simulink model "V0.2.4 - 2025-11-12 - FullFMS"  (R2025b)
settings: Solver=VariableStepAuto  StartTime=0.0  StopTime=inf  RelTol=1e-3
libraries: opcualib x2
(part 2 of 2)

== stateflow chart V0.2.4 - 2025-11-12 - FullFMS/Chart ==
  state VarDeclaration_20
    entry:
    %Control_20
    C_24_CRoute_In  = Control_20(1);
    C_25_CRoute_In  = Control_20(2);
    C_26_CRoute_In  = Control_20(3);
    C_27_CRoute_In  = Control_20(4);
    C_28_CRoute_In  = Control_20(5);
    C_29_CRoute_In  = Control_20(6);
    C_24_Request    = Control_20(7);
    C_24_CartDel    = Control_20(8);
    C_24_CRoute_Out = Control_20(9);
    C_25_Request    = Control_20(10);
    C_25_CartDel    = Control_20(11);
    C_25_CRoute_Out = Control_20(12);
    C_26_Request    = Control_20(13);
    C_26_CartDel    = Control_20(14);
    C_26_CRoute_Out = Control_20(15);
    C_27_Request    = Control_20(16);
    C_27_CartDel    = Control_20(17);
    C_27_CRoute_Out = Control_20(18);
    C_28_Request    = Control_20(19);
    C_28_CartDel    = Control_20(20);
    C_28_CRoute_Out = Control_20(21);
    C_29_Request    = Control_20(22);
    C_29_CartDel    = Control_20(23);
    C_29_CRoute_Out = Control_20(24);
    %Actuators_20
    F_22_Led_On       = Actuators_20(1);
    F_22_Led_Off      = Actuators_20(2);
    F_22_Conveyor   = Actuators_20(3);
    F_24_Release_FB   = Actuators_20(4);
    F_25_Release_FB   = Actuators_20(5);
    F_26_Release_FB   = Actuators_20(6);
    F_27_Release_FB   = Actuators_20(7);
    F_28_Release_FB   = Actuators_20(8);
    F_29_Release_FB   = Actuators_20(9);
    %Sensors_20
    O_20_On            = Sensors_20(1);
    O_20_Off           = Sensors_20(2);
    O_20_Controler_On  = Sensors_20(3);
    O_24_Cart_Stat     = Sensors_20(4);
    O_24_Cart_Next     = Sensors_20(5);
    O_24_Optic         = Sensors_20(6);
    O_24_Count         = Sensors_20(7);
    O_24_Pist_Bck      = Sensors_20(8);
    O_25_Cart_Stat     = Sensors_20(9);
    O_25_Cart_Next     = Sensors_20(10);
    O_25_Optic         = Sensors_20(11);
    O_25_Count         = Sensors_20(12);
    O_25_Pist_Back     = Sensors_20(13);
    O_26_Cart_Stat     = Sensors_20(14);
    O_26_Cart_Next     = Sensors_20(15);
    O_26_Optic         = Sensors_20(16);
    O_26_Count         = Sensors_20(17);
    O_26_Pist_Back     = Sensors_20(18);
    O_27_Cart_Stat     = Sensors_20(19);
    O_27_Cart_Next     = Sensors_20(20);
    O_27_Optic         = Sensors_20(21);
    O_27_Count         = Sensors_20(22);
    O_27_Pist_Back     = Sensors_20(23);
    O_28_Cart_Stat     = Sensors_20(24);
    O_28_Cart_Next     = Sensors_20(25);
    O_28_Optic         = Sensors_20(26);
    O_28_Count         = Sensors_20(27);
    O_28_Pist_Back     = Sensors_20(28);
    O_29_Cart_Stat     = Sensors_20(29);
    O_29_Cart_Next     = Sensors_20(30);
    O_29_Optic         = Sensors_20(31);
    O_29_Count         = Sensors_20(32);
    O_29_Pist_Back     = Sensors_20(33);
  state VarDeclaration_30
    entry:
    %AS_i_30
    A_34_Request    = AS_i_30(1);
    A_34_No_Cart    = AS_i_30(2);
    A_34_Cart_Full  = AS_i_30(3);
    A_34_CRoute_Out = AS_i_30(4);
    A_32_RoboCartID = AS_i_30(5);
    A_34_Cart_Stat  = AS_i_30(6);
    A_34_Cart_Next  = AS_i_30(7);
    A_34_Optic      = AS_i_30(8);
    A_34_Count      = AS_i_30(9);
    A_34_Pist_Bck   = AS_i_30(10);
    A_34_Release_FB = AS_i_30(11);
    A_34_CRoute_In  = AS_i_30(12);
    %Control_30
    C_30_Robot1   = Control_30(1);
    C_30_Robot2   = Control_30(2);
    C_35_Part_Del = Control_30(3);
    %Actuators_30
    F_33_Led_Start  = Actuators_30(1);
    F_33_Led_Reset  = Actuators_30(2);
    F_33_Led_Extra1 = Actuators_30(3);
    F_33_Led_Extra2 = Actuators_30(4);
    F_33_Spring_Cyl = Actuators_30(5);
    F_33_Cover_Cyl  = Actuators_30(6);
    %Sensors_30
    O_31_Start        = Sensors_30(1);
    O_31_Stop         = Sensors_30(2);
    O_31_Reset        = Sensors_30(3);
    O_31_Part_in_Claw = Sensors_30(4);
    O_31_Orientation  = Sensors_30(5);
    O_32_Sp_Cyl_Bck   = Sensors_30(6);
    O_32_Sp_Cyl_Fwd   = Sensors_30(7);
    O_32_Co_Cyl_Bck   = Sensors_30(8);
    O_32_Co_Cyl_Fwd   = Sensors_30(9);
    O_32_Sp_PickUp    = Sensors_30(10);
    O_32_Co_PickUp    = Sensors_30(11);
    O_32_CoMag_Empty  = Sensors_30(12);
  state VarDeclaration_40
    entry:
    %AS_i_40
    %Control_40
    %Actuators_40
    %Sensors_40
  state VarDeclaration_50
    entry:
    %AS_i_50
    A_54_Request    = AS_i_50(1);
    A_54_No_Cart    = AS_i_50(2);
    A_54_Cart_Full  = AS_i_50(3);
    A_54_CRoute_Out = AS_i_50(4);
    A_53_SortCartID = AS_i_50(5);
    A_54_Cart_Stat  = AS_i_50(6);
    A_54_Cart_Next  = AS_i_50(7);
    A_54_Optic      = AS_i_50(8);
    A_54_Count      = AS_i_50(9);
    A_54_Pist_Bck   = AS_i_50(10);
    A_54_Release_FB = AS_i_50(11);
    A_54_CRoute_In  = AS_i_50(12);
    C_55_Start      = AS_i_50(13);
    C_55_Cart2Del   = AS_i_50(14);
    %Control_50
    C_55_Initialization = Control_50(1);
    C_55_PD_Sort        = Control_50(2);
    C_52_Profibus       = Control_50(3);
    C_55_Start          = Control_50(4);
    C_55_Cart2Del       = Control_50(5);
    %Actuators_50
    F_52_Claw_2_Del  = Actuators_50(1);
    F_52_Claw_2_Cart = Actuators_50(2);
    F_52_Claw_Down   = Actuators_50(3);
    F_52_Close_Claw  = Actuators_50(4);
    F_53_Led_Start   = Actuators_50(5);
    F_53_Led_Reset   = Actuators_50(6);
    F_53_Led_Extra1  = Actuators_50(7);
    F_53_Led_Extra2  = Actuators_50(8);
    F_53_Panel_O4    = Actuators_50(9);
    F_53_Panel_O5    = Actuators_50(10);
    F_53_Panel_O6    = Actuators_50(11);
    F_53_Panel_O7    = Actuators_50(12);
    %Sensors_50
    O_50_Part_Reserve = Sensors_50(1);
    O_50_Claw_Cart    = Sensors_50(2);
    O_50_Claw_Del     = Sensors_50(3);
    O_50_Claw_Reserve = Sensors_50(4);
    O_50_Claw_Low     = Sensors_50(5);
    O_50_Claw_High    = Sensors_50(6);
    O_50_Part_in_Claw = Sensors_50(7);
    O_51_Start        = Sensors_50(8);
    O_51_Stop         = Sensors_50(9);
    O_51_Key_Pos      = Sensors_50(10);
    O_51_Reset        = Sensors_50(11);
    O_51_Panel_I4     = Sensors_50(12);
    O_51_Panel_I5     = Sensors_50(13);
    O_51_Panel_I6     = Sensors_50(14);
    O_51_Panel_I7     = Sensors_50(15);
  state VarDeclaration_60
    entry:
    %Control_60
    C_65_Initialization = Control_60(1);
    C_65_ID_1           = Control_60(2);
    C_65_ID_2           = Control_60(3);
    C_62_Profibus       = Control_60(4);
    C_65_RBS_Output     = Control_60(5);
    C_65_RSB_Output     = Control_60(6);
    C_65_BRS_Output     = Control_60(7);
    C_65_BSR_Output     = Control_60(8);
    C_65_SRB_Output     = Control_60(9);
    C_65_SBR_Output     = Control_60(10);
    %Actuators_60
    F_62_Conveyor   = Actuators_60(1);
    F_62_P1         = Actuators_60(2);
    F_62_P2         = Actuators_60(3);
    F_62_Identify   = Actuators_60(4);
    F_63_Led_Start  = Actuators_60(5);
    F_63_Led_Reset  = Actuators_60(6);
    F_63_Led_Extra1 = Actuators_60(7);
    F_63_Led_Extra2 = Actuators_60(8);
    F_63_Panel_O4   = Actuators_60(9);
    F_63_Panel_O5   = Actuators_60(10);
    F_63_Panel_O6   = Actuators_60(11);
    F_63_Panel_O7   = Actuators_60(12);
    %Sensors_60
    O_60_SPart      = Sensors_60(1);
    O_60_Slnd       = Sensors_60(2);
    O_60_SPhoto     = Sensors_60(3);
    O_60_Part_Pass  = Sensors_60(4);
    O_60_SL1_Bck    = Sensors_60(5);
    O_60_SL1_Fwd    = Sensors_60(6);
    O_60_SL2_Bck    = Sensors_60(7);
    O_60_SL2_Fwd    = Sensors_60(8);
    O_61_Start      = Sensors_60(9);
    O_61_Stop       = Sensors_60(10);
    O_61_Key_Pos    = Sensors_60(11);
    O_61_Reset      = Sensors_60(12);
    O_61_Panel_I4   = Sensors_60(13);
    O_61_Panel_I5   = Sensors_60(14);
    O_61_Panel_I6   = Sensors_60(15);
    O_61_Panel_I7   = Sensors_60(16);
  state VarDeclaration_70
    entry:
    %AS_i_70
    A_74_Request = AS_i_70(1);
    A_74_No_Cart = AS_i_70(2);
    A_74_Cart_Full = AS_i_70(3);
    A_74_CRoute_Out = AS_i_70(4);
    A_74_CRoute_In80 = AS_i_70(5);
    A_73_TestCartID = AS_i_70(6);
    A_74_Cart_Stat = AS_i_70(7);
    A_74_Cart_Next = AS_i_70(8);
    A_74_Optic = AS_i_70(9);
    A_74_Count = AS_i_70(10);
    A_74_Pist_Bck = AS_i_70(11);
    A_74_Release_FB = AS_i_70(12);
    A_74_CRoute_In = AS_i_70(13);
    %Control_70
    C_75_Initialization = Control_70(1);
    C_75_ID_Delivery1 = Control_70(2);
    C_75_ID_Delivery2 = Control_70(3);
    C_75_Part_Del = Control_70(4);
    C_75_RQ_Part_Del = Control_70(5);
    C_75_RQ_Wrong = Control_70(6);
    C_75_Identified80 = Control_70(7);
    C_75_Requested80 = Control_70(8);
    C_72_Profibus = Control_70(9);
    C_75_RQ_Delivery1 = Control_70(10);
    C_75_RQ_Delivery2 = Control_70(11);
    C_75_Identified = Control_70(12);
    C_75_Requested = Control_70(13);
    %Actuators_70
    F_72_Elev_Down = Actuators_70(1);
    F_72_Elev_Up = Actuators_70(2);
    F_72_Eject_Part = Actuators_70(3);
    F_72_Air_On = Actuators_70(4);
    F_73_Led_Start = Actuators_70(5);
    F_73_Led_Reset = Actuators_70(6);
    F_73_Led_Extra1 = Actuators_70(7);
    F_73_Led_Extra2 = Actuators_70(8);
    F_73_Panel_O4 = Actuators_70(9);
    F_73_Panel_O5 = Actuators_70(10);
    F_73_Panel_O6 = Actuators_70(11);
    F_73_Panel_O7 = Actuators_70(12);
    %Sensors_70
    O_70_SInductive = Sensors_70(1);
    O_70_SPart = Sensors_70(2);
    O_70_SStation = Sensors_70(3);
    O_70_SPart_Height = Sensors_70(4);
    O_70_Elev_High = Sensors_70(5);
    O_70_Elev_Low = Sensors_70(6);
    O_70_Pist_Back = Sensors_70(7);
    O_71_Start = Sensors_70(8);
    O_71_Stop = Sensors_70(9);
    O_71_Key_Pos = Sensors_70(10);
    O_71_Reset = Sensors_70(11);
    O_71_Panel_I4 = Sensors_70(12);
    O_71_Panel_I5 = Sensors_70(13);
    O_71_Panel_I6 = Sensors_70(14);
    O_71_Panel_I7 = Sensors_70(15);
  state VarDeclaration_80
    entry:
    %Control_80
    C_85_Initialization = Control_80(1);
    C_85_Part_Del = Control_80(2);
    C_82_Profibus = Control_80(3);
    C_83_RQ_Parts = Control_80(4);
    C_85_Start = Control_80(5);
    C_85_Single = Control_80(6);
    C_85_Continuous = Control_80(7);
    C_85_Counted = Control_80(8);
    %Actuators_80
    F_82_Pist_Adv = Actuators_80(1);
    F_82_Suction_On = Actuators_80(2);
    F_82_Suction_Off = Actuators_80(3);
    F_82_Arm_2_Del = Actuators_80(4);
    F_82_Arm_2_Mag = Actuators_80(5);
    F_83_Led_Start = Actuators_80(6);
    F_83_Led_Reset = Actuators_80(7);
    F_83_Led_Extra1 = Actuators_80(8);
    F_83_Led_Extra2 = Actuators_80(9);
    F_83_Panel_O4 = Actuators_80(10);
    F_83_Panel_O5 = Actuators_80(11);
    F_83_Panel_O6 = Actuators_80(12);
    F_83_Panel_O7 = Actuators_80(13);
    %Sensors_80
    O_80_Mag_Full = Sensors_80(1);
    O_80_Pist_Back = Sensors_80(2);
    O_80_Pist_Fwd = Sensors_80(3);
    O_80_Part_Stuck = Sensors_80(4);
    O_80_Arm_Mag = Sensors_80(5);
    O_80_Arm_Del = Sensors_80(6);
    O_80_Mag_Empty = Sensors_80(7);
    O_81_Start = Sensors_80(8);
    O_81_Stop = Sensors_80(9);
    O_81_Key_Pos = Sensors_80(10);
    O_81_Reset = Sensors_80(11);
    O_81_Panel_I4 = Sensors_80(12);
    O_81_Panel_I5 = Sensors_80(13);
    O_81_Panel_I6 = Sensors_80(14);
    O_81_Panel_I7 = Sensors_80(15);
  state VarDeclaration_90
    entry:
    %AS_i_90
    A_94_Request    = AS_i_90(1);
    A_94_No_Cart    = AS_i_90(2);
    A_94_Cart_Full  = AS_i_90(3);
    A_94_CRoute_Out = AS_i_90(4);
    A_93_ProcCartID = AS_i_90(5);
    A_94_Cart_Stat  = AS_i_90(6);
    A_94_Cart_Next  = AS_i_90(7);
    A_94_Optic      = AS_i_90(8);
    A_94_Count      = AS_i_90(9);
    A_94_Pist_Bck   = AS_i_90(10);
    A_94_Release_FB = AS_i_90(11);
    A_94_CRoute_In  = AS_i_90(12);
    %Control_90
    C_95_Initialization = Control_90(1);
    C_95_PD_Proc        = Control_90(2);
    C_95_PD_Cart        = Control_90(3);
    C_92_Profibus       = Control_90(4);
    C_95_Start          = Control_90(5);
    C_95_Cart2Del       = Control_90(6);
    C_95_Del2Cart       = Control_90(7);
    %Actuators_90
    F_92_Claw_2_Cart = Actuators_90(1);
    F_92_Claw_2_Del  = Actuators_90(2);
    F_92_Claw_Down   = Actuators_90(3);
    F_92_Close_Claw  = Actuators_90(4);
    F_93_Led_Start   = Actuators_90(5);
    F_93_Led_Reset   = Actuators_90(6);
    F_93_Led_Extra1  = Actuators_90(7);
    F_93_Led_Extra2  = Actuators_90(8);
    F_93_Panel_O4    = Actuators_90(9);
    F_93_Panel_O5    = Actuators_90(10);
    F_93_Panel_O6    = Actuators_90(11);
    F_93_Panel_O7    = Actuators_90(12);
    %Sensors_90
    O_90_Part_Reserve = Sensors_90(1);
    O_90_Claw_Del     = Sensors_90(2);
    O_90_Claw_Cart    = Sensors_90(3);
    O_90_Claw_Reserve = Sensors_90(4);
    O_90_Claw_Low     = Sensors_90(5);
    O_90_Claw_High    = Sensors_90(6);
    O_90_Part_in_Claw = Sensors_90(7);
    O_91_Start        = Sensors_90(8);
    O_91_Stop         = Sensors_90(9);
    O_91_Key_Pos      = Sensors_90(10);
    O_91_Reset        = Sensors_90(11);
    O_91_Panel_I4     = Sensors_90(12);
    O_91_Panel_I5     = Sensors_90(13);
    O_91_Panel_I6     = Sensors_90(14);
    O_91_Panel_I7     = Sensors_90(15);
  state VarDeclaration_100
    entry:
    %Control_100
    C_105_Initialization = Control_100(1);
    C_105_Part_ready     = Control_100(2);
    C_105_Test_Ok        = Control_100(3);
    C_105_Test_Fail      = Control_100(4);
    C_102_Profibus       = Control_100(5);
    C_103_RQ_Turns       = Control_100(6);
    C_105_Start          = Control_100(7);
    C_105_Test           = Control_100(8);
    C_105_TestDrill      = Control_100(9);
    C_105_Rotation       = Control_100(10);
    %Actuators_100
    F_102_Drill_On   = Actuators_100(1);
    F_102_RT_On      = Actuators_100(2);
    F_102_Drill_Down = Actuators_100(3);
    F_102_Drill_Up   = Actuators_100(4);
    F_102_Drill_Pin  = Actuators_100(5);
    F_102_Test_Pin   = Actuators_100(6);
    F_103_Led_Start  = Actuators_100(7);
    F_103_Led_Reset  = Actuators_100(8);
    F_103_Led_Extra1 = Actuators_100(9);
    F_103_Led_Extra2 = Actuators_100(10);
    F_103_Panel_O4   = Actuators_100(11);
    F_103_Panel_O5   = Actuators_100(12);
    F_103_Panel_O6   = Actuators_100(13);
    F_103_Panel_O7   = Actuators_100(14);
    %Sensors_100
    O_100_PInit_Pos   = Sensors_100(1);
    O_100_PDrill_Pos  = Sensors_100(2);
    O_100_PTest_Pos   = Sensors_100(3);
    O_100_SDrill_High = Sensors_100(4);
    O_100_SDrill_Low  = Sensors_100(5);
    O_100_RT_Sensor   = Sensors_100(6);
    O_100_PTest_Ok    = Sensors_100(7);
    O_101_Start       = Sensors_100(8);
    O_101_Stop        = Sensors_100(9);
    O_101_Key_Pos     = Sensors_100(10);
    O_101_Reset       = Sensors_100(11);
    O_101_Panel_I4    = Sensors_100(12);
    O_101_Panel_I5    = Sensors_100(13);
    O_101_Panel_I6    = Sensors_100(14);
    O_101_Panel_I7    = Sensors_100(15);
  state Distribution_Single
    state InitialCondition
      during:
      O_70_SSTation
      C_75_RQ_Wrong
      A_74_Croute_In80
      C_85_Single
      C_85_Start
      C_85_Part_Del
      C_86_Mag_Parts
      F_82_Pist_Adv
      F_82_Arm_2_Del
      F_82_Arm_2_Mag
      F_82_Suction_On
      F_82_Suction_Off
      F_83_Led_Extra1
      O_80_Arm_Mag
      O_80_Arm_Del
      O_80_Pist_Back
      O_80_Pist_Fwd
      O_80_Part_Stuck
      O_81_Start
      O_81_Key_Pos
      if ~O_70_SSTation && ...
      ~C_75_RQ_Wrong && ...
      ~A_74_Croute_In80 && ...
      C_85_Single && ...
      ~C_85_Start && ...
      ~C_85_Part_Del && ...
      C_86_Mag_Parts ~= 0 && ...
      ~F_82_Pist_Adv && ...
      ~F_82_Arm_2_Del && ...
      ~F_82_Arm_2_Mag && ...
      ~F_82_Suction_On && ...
      ~F_82_Suction_Off && ...
      ~F_83_Led_Extra1 && ...
      O_80_Arm_Mag && ...
      ~O_80_Arm_Del && ...
      O_80_Pist_Back && ...
      ~O_80_Pist_Fwd && ...
      ~O_80_Part_Stuck && ...
      ~O_81_Start && ...
      O_81_Key_Pos
      status = true;
      else
      status = false;
      end
    state ArmToDelivery
      during:
      F_82_Arm_2_Del
      if F_82_Arm_2_Del
      status1 = true;
      else
      status1 = false;
      end
    state ArmArrives_FeedsPart
      during:
      F_82_Pist_Adv
      F_82_Arm_2_Del
      O_80_Arm_Del
      if F_82_Pist_Adv && ...
      ~F_82_Arm_2_Del && ...
      O_80_Arm_Del
      status3 = true;
      else
      status3 = false;
      end
    state PartFed
      during:
      C_86_Mag_Parts
      F_82_Pist_Adv
      O_80_Pist_Fwd
      if C_86_Mag_Parts ~= 0 && ...
      ~F_82_Pist_Adv && ...
      O_80_Pist_Fwd
      status5 = true;
      else
      status5 = false;
      end
    state ArmToMagazine
      during:
      F_82_Arm_2_Mag
      if F_82_Arm_2_Mag
      status7 = true;
      else
      status7 = false;
      end
    state ArmArrives_PicksPart
      during:
      F_82_Arm_2_Mag
      F_82_Suction_On
      if ~F_82_Arm_2_Mag && ...
      F_82_Suction_On
      status9 = true;
      else
      status9 = false;
      end
    state ArmToDelivery1
      during:
      F_82_Arm_2_Del
      if F_82_Arm_2_Del
      status10 = true;
      else
      status10 = false;
      end
    state ArmArrives_DeliversPart
      during:
      F_82_Arm_2_Del
      F_82_Suction_On
      F_82_Suction_Off
      if ~F_82_Arm_2_Del && ...
      ~F_82_Suction_On && ...
      F_82_Suction_Off
      status12 = true;
      else
      status12 = false;
      end
    state ArmToMagazine1
      during:
      C_85_Part_Del
      F_82_Arm_2_Mag
      F_82_Suction_Off
      F_83_Led_Extra1
      if C_85_Part_Del && ...
      ~F_82_Arm_2_Mag && ...
      ~F_82_Suction_Off && ...
      F_83_Led_Extra1
      status13 = true;
      else
      status13 = false;
      end
    state ArmArrives_Finish
      during:
      F_82_Arm_2_Mag
    state ArmCloseDelivery
      during:
      O_70_SSTation
      if O_70_SSTation
      status2 = true;
      else
      status2 = false;
      end
    state PistonStartsMoveForward
      during:
      O_80_Pist_Back
      if ~O_80_Pist_Back
      status4 = true;
      else
      status4 = false;
      end
    state PistonStartsMoveBackward
      during:
      O_80_Pist_Fwd
      if ~O_80_Pist_Fwd
      status6 = true;
      else
      status6 = false;
      end
    state ArmCloseDeliver1
      during:
      O_70_SSTation
      if ~O_70_SSTation
      status8 = true;
      else
      status8 = false;
      end
    state ArmCloseDelivery2
      during:
      O_70_SSTation
      if O_70_SSTation
      status11 = true;
      else
      status11 = false;
      end
    state ArmCloseDeliver3
      during:
      O_70_SSTation
      if ~O_70_SSTation
      status14 = true;
      else
      status14 = false;
      end
    state T1
      during:
      C_85_Part_Del
      F_83_Led_Extra1
    (default) -> Distribution_Single.InitialCondition
    Distribution_Single.ArmArrives_DeliversPart -> Distribution_Single.ArmToMagazine1 : [O_80_Part_Stuck == false && ...
        | status12 == true]
    Distribution_Single.ArmToMagazine -> Distribution_Single.ArmArrives_PicksPart [order 2] : [O_80_Arm_Mag == true && ...
        | status8 == true]
    Distribution_Single.ArmToDelivery1 -> Distribution_Single.ArmArrives_DeliversPart [order 2] : [O_80_Arm_Del == true && ...
        | status11 == true]
    Distribution_Single.ArmToDelivery -> Distribution_Single.ArmArrives_FeedsPart [order 2] : [O_80_Arm_Del == true && ...
        | status2 == true]
    Distribution_Single.ArmArrives_PicksPart -> Distribution_Single.ArmToDelivery1 : [O_80_Part_Stuck == true && ...
        | status9 == true]
    Distribution_Single.ArmToMagazine1 -> Distribution_Single.ArmArrives_Finish [order 2] : [O_80_Arm_Mag == true && ...
        | status14 == true]
    Distribution_Single.ArmArrives_FeedsPart -> Distribution_Single.PartFed [order 2] : [O_80_Piston_Fwd == true && ...
        | status4 == true]
    Distribution_Single.PartFed -> Distribution_Single.ArmToMagazine [order 2] : [O_80_Piston_Back == true && ...
        | status6 == true]
    Distribution_Single.InitialCondition -> Distribution_Single.ArmToDelivery : [O_81_Start == true | ...
        | C_85_Start == true | ...
        | C_75_RQ_Wrong == true | ...
        | (A_74_Croute_In80 == true && O_81_Key_Pos == true) ]
    Distribution_Single.ArmToDelivery -> Distribution_Single.ArmCloseDelivery [order 1] : [O_80_Arm_Mag == false &&....
        |  status1 ==true]
    Distribution_Single.ArmToDelivery1 -> ArmCloseDelivery2 [order 1] : [O_80_Arm_Mag == false &&....
        |  status10 ==true]
    Distribution_Single.ArmArrives_FeedsPart -> Distribution_Single.PistonStartsMoveForward [order 1] : [status3 == true]
    Distribution_Single.PartFed -> Distribution_Single.PistonStartsMoveBackward [order 1] : [status5 == true]
    Distribution_Single.ArmToMagazine -> Distribution_Single.ArmCloseDeliver1 [order 1] : [O_80_Arm_Del == false &&....
        |  status7 ==true]
    Distribution_Single.ArmToMagazine1 -> (junction 650) [order 1]
    (junction 650) -> ArmCloseDeliver3 [order 1] : [O_80_Arm_Del == false &&....
        |  status13 ==true]
    (junction 650) -> Distribution_Single.T1 [order 2] : after(4,sec)
  state Start
    during:
    C_24_Request
  state CartToTesting
    state InitialCondition
      during:
      C_24_Request
      F_22_Conveyor
      F_29_Release_FB
      A_54_Release_FB
      A_53_SortCartID
      O_29_Pist_Back
      A_54_Pist_Bck
      O_29_Cart_Stat
      A_54_Cart_Stat
      A_54_No_Cart
      F_53_Led_Extra1
      O_29_Cart_Next
      A_54_Cart_Next
      A_73_TestCartID
      O_24_Cart_Stat
      A_74_Cart_Stat
      C_24_CartDel
      A_74_No_Cart
      F_73_Led_Extra1
      A_74_CRoute_In
      if ~C_24_Request && ...
      ~F_22_Conveyor && ...
      ~F_29_Release_FB && ...
      ~A_54_Release_FB && ...
      A_53_SortCartID ~= 0 && ...
      ~O_29_Pist_Back && ...
      ~A_54_Pist_Bck && ...
      O_29_Cart_Stat && ...
      A_54_Cart_Stat && ...
      ~A_54_No_Cart && ...
      ~F_53_Led_Extra1 && ...
      ~O_29_Cart_Next && ...
      ~A_54_Cart_Next && ...
      A_73_TestCartID == 0 && ...
      ~O_24_Cart_Stat && ...
      ~A_74_Cart_Stat && ...
      ~C_24_CartDel && ...
      A_74_No_Cart && ...
      F_73_Led_Extra1 && ...
      ~A_74_CRoute_In
      status = true;
      else
      status = false;
      end
    state StartsProcess
      during:
      C_24_Request
      F_22_Conveyor
      F_29_Release_FB
      A_54_Release_FB
      A_53_SortCartID
      O_29_Pist_Back
      A_54_Pist_Bck
      if C_24_Request && ...
      F_22_Conveyor && ...
      F_29_Release_FB && ...
      A_54_Release_FB && ...
      A_53_SortCartID == 0 && ...
      O_29_Pist_Back && ...
      A_54_Pist_Bck
      status2 = true;
      else
      status2 = false;
      end
    state CartStartsMoving
      during:
      O_29_Cart_Stat
      A_54_Cart_Stat
      A_54_No_Cart
      F_53_Led_Extra1
      if ~O_29_Cart_Stat && ...
      ~A_54_Cart_Stat && ...
      A_54_No_Cart && ...
      F_53_Led_Extra1
      status3 = true;
      else
      status3 = false;
      end
    state CartGetsNearNextStation
      during:
      F_29_Release_FB
      A_54_Release_FB
      O_29_Pist_Back
      A_54_Pist_Bck
      O_29_Cart_Next
      A_54_Cart_Next
      if ~F_29_Release_FB && ...
      ~A_54_Release_FB && ...
      ~O_29_Pist_Back && ...
      ~A_54_Pist_Bck && ...
      O_29_Cart_Next && ...
      A_54_Cart_Next
      status4 = true;
      else
      status4 = false;
      end
    state DetectionofCartNumberinStation
      during:
      A_73_TestCartID
      if ~A_73_TestCartID
      status5 = true;
      end
    state CartPassesNextStation
      during:
      O_29_Cart_Next
      A_54_Cart_Next
      if ~O_29_Cart_Next && ...
      ~A_54_Cart_Next
      status6 = true;
      else
      status6 = false;
      end
    state CartArrivesinNextStation
      during:
      O_24_Cart_Stat
      A_74_Cart_Stat
      C_24_CartDel
      A_74_No_Cart
      F_73_Led_Extra1
      A_74_CRoute_In
      if O_24_Cart_Stat &&...
      A_74_Cart_Stat &&...
      C_24_CartDel &&...
      ~A_74_No_Cart &&...
      ~F_73_Led_Extra1 &&...
      A_74_CRoute_In
      status7 = true;
      else
      status7 = false;
      end
    state T3
      during:
      C_24_CartDel
    state T2
      during:
      A_74_CRoute_In
    state T1
      during:
      C_24_Request
    (default) -> CartToTesting.InitialCondition
    CartStartsMoving -> CartGetsNearNextStation : [O_29_Cart_Next == true && ...
        | status3 == true]
    DetectionofCartNumberinStation -> CartPassesNextStation : [O_29_Cart_Next == false && ...
        | status5 == true]
    CartGetsNearNextStation -> DetectionofCartNumberinStation : [A_73_TestCartID == 0 && ...
        | status4 == true]
    CartPassesNextStation -> CartArrivesinNextStation : [O_24_Cart_Stat == true && ...
        | status6 == true]
    StartsProcess -> CartStartsMoving [order 1] : [O_29_Cart_Stat == false && ...
        |  status2 == true]
    CartToTesting.InitialCondition -> StartsProcess : [C_24_Request == true && ...
        |  status == true]
    CartArrivesinNextStation -> (junction 582)
    StartsProcess -> CartToTesting.T1 [order 2] : [after(2, sec)]
    (junction 582) -> T3 [order 2] : [after(3,sec)]
    (junction 582) -> T2 [order 1] : [after(2,sec)]
  state Distribution_Continuous
    state InitialCondition
      during:
      O_70_SSTation
      C_75_RQ_Wrong
      A_74_Croute_In80
      C_85_Single
      C_85_Start
      C_85_Part_Del
      C_86_Mag_Parts
      F_82_Pist_Adv
      F_82_Arm_2_Del
      F_82_Arm_2_Mag
      F_82_Suction_On
      F_82_Suction_Off
      F_83_Led_Extra1
      O_80_Arm_Mag
      O_80_Arm_Del
      O_80_Pist_Back
      O_80_Pist_Fwd
      O_80_Part_Stuck
      O_81_Start
      O_81_Key_Pos
      if ~O_70_SSTation && ...
      ~C_75_RQ_Wrong && ...
      ~A_74_Croute_In80 && ...
      C_85_Single && ...
      ~C_85_Start && ...
      ~C_85_Part_Del && ...
      C_86_Mag_Parts ~= 0 && ...
      ~F_82_Pist_Adv && ...
      ~F_82_Arm_2_Del && ...
      ~F_82_Arm_2_Mag && ...
      ~F_82_Suction_On && ...
      ~F_82_Suction_Off && ...
      ~F_83_Led_Extra1 && ...
      O_80_Arm_Mag && ...
      ~O_80_Arm_Del && ...
      O_80_Pist_Back && ...
      ~O_80_Pist_Fwd && ...
      ~O_80_Part_Stuck && ...
      ~O_81_Start && ...
      O_81_Key_Pos
      status = true;
      else
      status = false;
      end
    state ArmToDelivery
      during:
      F_82_Arm_2_Del
      if F_82_Arm_2_Del
      status1 = true;
      else
      status1 = false;
      end
    state ArmArrives_FeedsPart
      during:
      F_82_Pist_Adv
      F_82_Arm_2_Del
      O_80_Arm_Del
      if F_82_Pist_Adv && ...
      ~F_82_Arm_2_Del && ...
      O_80_Arm_Del
      status3 = true;
      else
      status3 = false;
      end
    state PartFed
      during:
      C_86_Mag_Parts
      F_82_Pist_Adv
      O_80_Pist_Fwd
      if C_86_Mag_Parts ~= 0 && ...
      ~F_82_Pist_Adv && ...
      O_80_Pist_Fwd
      status5 = true;
      else
      status5 = false;
      end
    state ArmToMagazine
      during:
      F_82_Arm_2_Mag
      if F_82_Arm_2_Mag
      status7 = true;
      else
      status7 = false;
      end
    state ArmArrives_PicksPart
      during:
      F_82_Arm_2_Mag
      F_82_Suction_On
      if ~F_82_Arm_2_Mag && ...
      F_82_Suction_On
      status9 = true;
      else
      status9 = false;
      end
    state ArmToDelivery1
      during:
      F_82_Arm_2_Del
      if F_82_Arm_2_Del
      status10 = true;
      else
      status10 = false;
      end
    state ArmArrives_DeliversPart
      during:
      F_82_Arm_2_Del
      F_82_Suction_On
      F_82_Suction_Off
      if ~F_82_Arm_2_Del && ...
      ~F_82_Suction_On && ...
      F_82_Suction_Off
      status12 = true;
      else
      status12 = false;
      end
    state PartDel_CheckLoop
      during:
      C_85_Part_Del
      F_82_Arm_2_Mag
      F_82_Suction_Off
      F_83_Led_Extra1
      if C_85_Part_Del && ...
      F_83_Led_Extra1 && ...
      C_86_Mag_Parts ~= 0
      LoopDistCont = true;
      else
      LoopDistCont = false;
      end
    state ArmToMagazine1
      during:
      F_82_Arm_2_Mag
      if F_82_Arm_2_Mag
      status12 = true;
      else
      status12 = false;
      end
    state ArmArrives_Finish
      during:
      F_82_Arm_2_Mag
    state ArmCloseDelivery
      during:
      O_70_SSTation
      if O_70_SSTation
      status2 = true;
      else
      status2 = false;
      end
    state PistonStartsMoveForward
      during:
      O_80_Pist_Back
      if ~O_80_Pist_Back
      status4 = true;
      else
      status4 = false;
      end
    state PistonStartsMoveBackward
      during:
      O_80_Pist_Fwd
      if ~O_80_Pist_Fwd
      status6 = true;
      else
      status6 = false;
      end
    state ArmCloseDeliver1
      during:
      O_70_SSTation
      if ~O_70_SSTation
      status8 = true;
      else
      status8 = false;
      end
    state ArmCloseDelivery3
      during:
      O_70_SSTation
      if O_70_SSTation
      status11 = true;
      else
      status11 = false;
      end
    state ArmCloseDeliver4
      during:
      O_70_SSTation
      if ~O_70_SSTation
      status14 = true;
      else
      status14 = false;
      end
    state T1
      during:
      C_85_Part_Del
      F_83_Led_Extra1
    (default) -> Distribution_Continuous.InitialCondition
    Distribution_Continuous.ArmToDelivery1 -> Distribution_Continuous.ArmArrives_DeliversPart [order 2] : [O_80_Arm_Del == true && ...
        | status11 == true]
    Distribution_Continuous.ArmArrives_DeliversPart -> PartDel_CheckLoop : [O_80_Part_Stuck == false && ...
        | status12 == true]
    Distribution_Continuous.ArmToMagazine -> Distribution_Continuous.ArmArrives_PicksPart [order 2] : [O_80_Arm_Mag == true && ...
        | status8 == true]
    Distribution_Continuous.ArmArrives_PicksPart -> Distribution_Continuous.ArmToDelivery1 : [O_80_Part_Stuck == true && ...
        | status9 == true]
    PartDel_CheckLoop -> Distribution_Continuous.ArmToMagazine1 [order 2] : [LoopDistCont == false]
    Distribution_Continuous.ArmToDelivery -> Distribution_Continuous.ArmArrives_FeedsPart [order 2] : [O_80_Arm_Del == true && ...
        | status2 == true]
    Distribution_Continuous.ArmToMagazine1 -> Distribution_Continuous.ArmArrives_Finish [order 1] : [O_80_Arm_Mag == true && ...
        | status14 == true]
    Distribution_Continuous.ArmArrives_FeedsPart -> Distribution_Continuous.PartFed [order 2] : [O_80_Piston_Fwd == true && ...
        | status4 == true]
    Distribution_Continuous.PartFed -> Distribution_Continuous.ArmToMagazine [order 2] : [O_80_Piston_Back == true && ...
        | status6 == true]
    Distribution_Continuous.InitialCondition -> Distribution_Continuous.ArmToDelivery : [O_81_Start == true | ...
        | C_85_Start == true | ...
        | C_75_RQ_Wrong == true | ...
        | (A_74_Croute_In80 == true && O_81_Key_Pos == true) ]
    Distribution_Continuous.ArmToDelivery -> Distribution_Continuous.ArmCloseDelivery [order 1] : [O_80_Arm_Mag == false &&....
        |  status1 ==true]
    (junction 708) -> Distribution_Continuous.ArmArrives_FeedsPart
    Distribution_Continuous.ArmToDelivery1 -> ArmCloseDelivery3 [order 1] : [O_80_Arm_Mag == false &&....
        |  status10 ==true]
    (junction 706) -> (junction 708)
    Distribution_Continuous.ArmArrives_FeedsPart -> Distribution_Continuous.PistonStartsMoveForward [order 1] : [status3 == true]
    Distribution_Continuous.PartFed -> Distribution_Continuous.PistonStartsMoveBackward [order 1] : [status5 == true]
    Distribution_Continuous.ArmToMagazine -> Distribution_Continuous.ArmCloseDeliver1 [order 1] : [O_80_Arm_Del == false &&....
        |  status7 ==true]
    PartDel_CheckLoop -> (junction 707) [order 1] : [LoopDistCont == true]
    PartDel_CheckLoop -> Distribution_Continuous.T1 [order 3] : after(4,sec)
    Distribution_Continuous.ArmToMagazine1 -> ArmCloseDeliver4 [order 2] : [O_80_Arm_Del == false &&....
        |  status13 ==true]
    (junction 707) -> (junction 706)
  state Test_Drill
    during:
    C_105_Part_ready
  state CartToHandling2
    during:
    C_25_CartDel
  state DeliverToProcessing
    during:
    C_95_PD_Proc
    C_105_TestDrill
    C_105_Test
    C_105_Rotation
  state Test_Only
    during:
    C_105_Part_ready
  state CarrinhoParaVision
    during:
    C_26_CartDel
  state ReturnToCart
    during:
    C_95_PD_Cart
  state Rotation_Only
    during:
    C_105_Part_ready
  state IdentifiesPart
    during:
    C_75_Part_Del
    A_74_CRoute_Out
  state Distribution_Counted
  (default) -> VarDeclaration_100
  VarDeclaration_40 -> VarDeclaration_30
  VarDeclaration_90 -> VarDeclaration_80
  VarDeclaration_100 -> VarDeclaration_90
  VarDeclaration_30 -> VarDeclaration_20
  VarDeclaration_80 -> VarDeclaration_70
  VarDeclaration_60 -> VarDeclaration_50
  VarDeclaration_50 -> VarDeclaration_40
  VarDeclaration_70 -> VarDeclaration_60
  VarDeclaration_20 -> Start
  (junction 729) -> Distribution_Single
  (junction 726) -> (junction 729) [order 2] : [C_85_Single]
  Distribution_Single -> IdentifiesPart : [C_85_Part_Del == true]
  Start -> CartToTesting : [C_24_Request == true]
  Test_Drill -> ReturnToCart : [C_105_Part_ready == true]
  (junction 573) -> Test_Drill [order 1] : [C_105_TestDrill == true]
  DeliverToProcessing -> (junction 573) : [C_95_PD_Proc == true]
  (junction 573) -> Test_Only [order 2] : [C_105_Test == true]
  IdentifiesPart -> CartToHandling2 : [C_75_Part_Del == true && A_74_CRoute_Out == true ]
  ReturnToCart -> CarrinhoParaVision : [C_95_PD_Cart == true]
  (junction 573) -> Rotation_Only [order 3] : [C_105_Rotation == true]
  Test_Only -> ReturnToCart : [C_105_Part_ready == true]
  CartToHandling2 -> DeliverToProcessing : [C_25_CartDel == true]
  Rotation_Only -> ReturnToCart : [C_105_Part_ready == true]
  CartToTesting -> (junction 726) : [C_24_CartDe]
  (junction 726) -> Distribution_Continuous [order 1] : [C_85_Continuous]
  (junction 726) -> (junction 732) [order 3] : [C_85_Counted]
  Distribution_Continuous -> IdentifiesPart : [C_85_Part_Del == true]
  (junction 732) -> Distribution_Counted
  data: Control_80 input; Actuators_80 input; Sensors_80 input; AS_i_70 input; Control_70 input; Actuators_70 input; Sensors_70 input; C_82_Profibus local; C_83_RQ_Parts local; C_85_Continuous local; C_85_Counted local; C_85_Initialization local; C_85_Part_Del local; C_85_Single local; C_85_Start local; F_82_Arm_2_Del local; F_82_Arm_2_Mag local; F_82_Pist_Adv local; F_82_Suction_Off local; F_82_Suction_On local; F_83_Led_Extra1 local; F_83_Led_Extra2 local; F_83_Led_Reset local; F_83_Led_Start local; F_83_Panel_O4 local; F_83_Panel_O5 local; F_83_Panel_O6 local; F_83_Panel_O7 local; O_80_Arm_Del local; O_80_Arm_Mag local; O_80_Mag_Empty local; O_80_Mag_Full local; O_80_Part_Stuck local; O_80_Pist_Back local; O_80_Pist_Fwd local; O_81_Key_Pos local; O_81_Panel_I4 local; O_81_Panel_I5 local; O_81_Panel_I6 local; O_81_Panel_I7 local; O_81_Reset local; O_81_Start local; O_81_Stop local; C_75_ID_Delivery1 local; C_75_ID_Delivery2 local; C_75_Identified local; C_75_Identified80 local; C_75_Initialization local; C_75_Part_Del local; C_75_RQ_Delivery1 local; C_75_RQ_Delivery2 local; C_75_RQ_Part_Del local; C_75_RQ_Wrong local; C_75_Requested local; C_75_Requested80 local; F_72_Air_On local; F_72_Eject_Part local; F_72_Elev_Down local; F_72_Elev_Up local; F_73_Led_Extra1 local; F_73_Led_Extra2 local; F_73_Led_Reset local; F_73_Led_Start local; F_73_Panel_O4 local; F_73_Panel_O5 local; F_73_Panel_O6 local; F_73_Panel_O7 local; O_70_Elev_High local; O_70_Elev_Low local; O_70_Pist_Back local; O_70_SInductive local; O_70_SPart local; O_70_SPart_Height local; O_70_SStation local; O_71_Key_Pos local; O_71_Panel_I4 local; O_71_Panel_I5 local; O_71_Panel_I6 local; O_71_Panel_I7 local; O_71_Reset local; O_71_Start local; O_71_Stop local; A_73_TestCartID local; A_74_CRoute_In local; A_74_CRoute_In80 local; A_74_CRoute_Out local; A_74_Cart_Full local; A_74_Cart_Next local; A_74_Cart_Stat local; A_74_Count local; A_74_No_Cart local; A_74_Optic local; A_74_Pist_Bck local; A_74_Release_FB local; A_74_Request local; C_72_Profibus local; AS_i_30 input; AS_i_50 input; AS_i_90 input; Actuators_100 input; Actuators_20 input; Actuators_30 input; Actuators_50 input; Actuators_60 input; Actuators_90 input; Control_100 input; Control_20 input; Control_30 input; Control_50 input; Control_60 input; Control_90 input; Sensors_100 input; Sensors_20 input; Sensors_30 input; Sensors_50 input; Sensors_60 input; Sensors_90 input; A_32_RoboCartID local; A_34_CRoute_In local; A_34_CRoute_Out local; A_34_Cart_Full local; A_34_Cart_Next local; A_34_Cart_Stat local; A_34_Count local; A_34_No_Cart local; A_34_Optic local; A_34_Pist_Bck local; A_34_Release_FB local; A_34_Request local; A_53_SortCartID local; A_54_CRoute_In local; A_54_CRoute_Out local; A_54_Cart_Full local; A_54_Cart_Next local; A_54_Cart_Stat local; A_54_Count local; A_54_No_Cart local; A_54_Optic local; A_54_Pist_Bck local; A_54_Release_FB local; A_54_Request local; A_93_ProcCartID local; A_94_CRoute_In local; A_94_CRoute_Out local; A_94_Cart_Full local; A_94_Cart_Next local; A_94_Cart_Stat local; A_94_Count local; A_94_No_Cart local; A_94_Optic local; A_94_Pist_Bck local; A_94_Release_FB local; A_94_Request local; C_102_Profibus local; C_103_RQ_Turns local; C_105_Initialization local; C_105_Part_ready local; C_105_Rotation local; C_105_Start local; C_105_Test local; C_105_TestDrill local; C_105_Test_Fail local; C_105_Test_Ok local; C_24_CRoute_In local; C_24_CRoute_Out local; C_24_CartDel local; C_24_Request local; C_25_CRoute_In local; C_25_CRoute_Out local; C_25_CartDel local; C_25_Request local; C_26_CRoute_In local; C_26_CRoute_Out local; C_26_CartDel local; C_26_Request local; C_27_CRoute_In local; C_27_CRoute_Out local; C_27_CartDel local; C_27_Request local; C_28_CRoute_In local; C_28_CRoute_Out local; C_28_CartDel local; C_28_Request local; C_29_CRoute_In local; C_29_CRoute_Out local; C_29_CartDel local; C_29_Request local; C_30_Robot1 local; C_30_Robot2 local; C_35_Part_Del local; C_52_Profibus local; C_55_Cart2Del local; C_55_Initialization local; C_55_PD_Sort local; C_55_Start local; C_62_Profibus local; C_65_BRS_Output local; C_65_BSR_Output local; C_65_ID_1 local; C_65_ID_2 local; C_65_Initialization local; C_65_RBS_Output local; C_65_RSB_Output local; C_65_SBR_Output local; C_65_SRB_Output local; C_92_Profibus local; C_95_Cart2Del local; C_95_Del2Cart local; C_95_Initialization local; C_95_PD_Cart local; C_95_PD_Proc local; C_95_Start local; F_102_Drill_Down local; F_102_Drill_On local; F_102_Drill_Pin local; F_102_Drill_Up local; F_102_RT_On local; F_102_Test_Pin local; F_103_Led_Extra1 local; F_103_Led_Extra2 local; F_103_Led_Reset local; F_103_Led_Start local; F_103_Panel_O4 local; F_103_Panel_O5 local; F_103_Panel_O6 local; F_103_Panel_O7 local; F_22_Led_Off local; F_22_Led_On local; F_24_Release_FB local; F_25_Release_FB local; F_26_Release_FB local; F_27_Release_FB local; F_28_Release_FB local; F_29_Release_FB local; F_33_Cover_Cyl local; F_33_Led_Extra1 local; F_33_Led_Extra2 local; F_33_Led_Reset local; F_33_Led_Start local; F_33_Spring_Cyl local; F_52_Claw_2_Cart local; F_52_Claw_2_Del local; F_52_Claw_Down local; F_52_Close_Claw local; F_53_Led_Extra1 local; F_53_Led_Extra2 local; F_53_Led_Reset local; F_53_Led_Start local; F_53_Panel_O4 local; F_53_Panel_O5 local; F_53_Panel_O6 local; F_53_Panel_O7 local; F_62_Conveyor local; F_62_Identify local; F_62_P1 local; F_62_P2 local; F_63_Led_Extra1 local; F_63_Led_Extra2 local; F_63_Led_Reset local; F_63_Led_Start local; F_63_Panel_O4 local; F_63_Panel_O5 local; F_63_Panel_O6 local; F_63_Panel_O7 local; F_92_Claw_2_Cart local; F_92_Claw_2_Del local; F_92_Claw_Down local; F_92_Close_Claw local; F_93_Led_Extra1 local; F_93_Led_Extra2 local; F_93_Led_Reset local; F_93_Led_Start local; F_93_Panel_O4 local; F_93_Panel_O5 local; F_93_Panel_O6 local; F_93_Panel_O7 local; O_100_PDrill_Pos local; O_100_PInit_Pos local; O_100_PTest_Ok local; O_100_PTest_Pos local; O_100_RT_Sensor local; O_100_SDrill_High local; O_100_SDrill_Low local; O_101_Key_Pos local; O_101_Panel_I4 local; O_101_Panel_I5 local; O_101_Panel_I6 local; O_101_Panel_I7 local; O_101_Reset local; O_101_Start local; O_101_Stop local; O_20_Controler_On local; O_20_Off local; O_20_On local; O_24_Cart_Next local; O_24_Cart_Stat local; O_24_Count local; O_24_Optic local; O_24_Pist_Bck local; O_25_Cart_Next local; O_25_Cart_Stat local; O_25_Count local; O_25_Optic local; O_25_Pist_Back local; O_26_Cart_Next local; O_26_Cart_Stat local; O_26_Count local; O_26_Optic local; O_26_Pist_Back local; O_27_Cart_Next local; O_27_Cart_Stat local; O_27_Count local; O_27_Optic local; O_27_Pist_Back local; O_28_Cart_Next local; O_28_Cart_Stat local; O_28_Count local; O_28_Optic local; O_28_Pist_Back local; O_29_Cart_Next local; O_29_Cart_Stat local; O_29_Count local; O_29_Optic local; O_29_Pist_Back local; O_31_Orientation local; O_31_Part_in_Claw local; O_31_Reset local; O_31_Start local; O_31_Stop local; O_32_CoMag_Empty local; O_32_Co_Cyl_Bck local; O_32_Co_Cyl_Fwd local; O_32_Co_PickUp local; O_32_Sp_Cyl_Bck local; O_32_Sp_Cyl_Fwd local; O_32_Sp_PickUp local; O_50_Claw_Cart local; O_50_Claw_Del local; O_50_Claw_High local; O_50_Claw_Low local; O_50_Claw_Reserve local; O_50_Part_Reserve local; O_50_Part_in_Claw local; O_51_Key_Pos local; O_51_Panel_I4 local; O_51_Panel_I5 local; O_51_Panel_I6 local; O_51_Panel_I7 local; O_51_Reset local; O_51_Start local; O_51_Stop local; O_60_Part_Pass local; O_60_SL1_Bck local; O_60_SL1_Fwd local; O_60_SL2_Bck local; O_60_SL2_Fwd local; O_60_SPart local; O_60_SPhoto local; O_60_Slnd local; O_61_Key_Pos local; O_61_Panel_I4 local; O_61_Panel_I5 local; O_61_Panel_I6 local; O_61_Panel_I7 local; O_61_Reset local; O_61_Start local; O_61_Stop local; O_90_Claw_Cart local; O_90_Claw_Del local; O_90_Claw_High local; O_90_Claw_Low local; O_90_Claw_Reserve local; O_90_Part_Reserve local; O_90_Part_in_Claw local; O_91_Key_Pos local; O_91_Panel_I4 local; O_91_Panel_I5 local; O_91_Panel_I6 local; O_91_Panel_I7 local; O_91_Reset local; O_91_Start local; O_91_Stop local; F_22_Conveyor local; status6 local; status local; status2 local; status3 local; status4 local; status5 local; status7 local; A_74_Croute_In80 input; status1 local; O_70_SSTation input; O_70_SSTantion input; C_86_Mag_Parts input; O_80_Piston_Back input; O_80_Piston_Fwd input; status10 local; status11 local; status12 local; status13 local; status9 local; status8 local; status14 local; LoopDistCont local
